simulink model "power_microgrid_v5_battery"  (R2018b)
settings: Solver=ode23tb  StartTime=0.0  StopTime=24*60*60  FixedStep=1/(1000)  MaxStep=60  RelTol=1e-4
PreLoadFcn:
  | load('solar_load_data_24h.mat')
PostLoadFcn:
  | data = xlsread('Domestic_data_all_x3','Sheet1');
  | breakpoints1 = data(2:end,1)'
  | breakpoints2 = data(1,2:end)
  | table_data = data(2:end,2:end)
values from neighbouring files (symbols this model uses):
  SPD_1min = [0 0 0 0 0 0 0 0 0 0 0 0 ... (1441 elements, 1441x1)]    [default_PV_data.mat]
  SPT_1min = [0 60 120 180 240 300 360 420 480 540 600 660 ... (1441 elements, 1441x1)]    [default_PV_data.mat]
libraries: powerlib x155
(part 2 of 5)

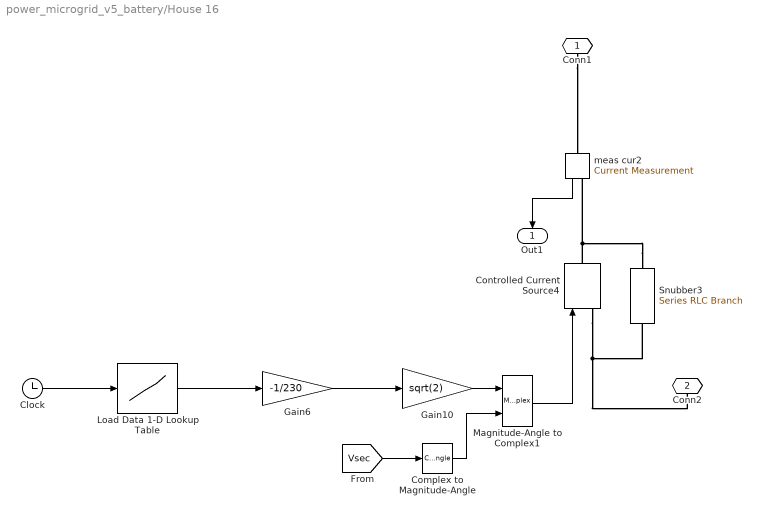
== system power_microgrid_v5_battery/House 16 ==
  Clock : Clock
  Complex to Magnitude-Angle : ComplexToMagnitudeAngle  Output=Angle
  Controlled Current Source4 : powerlib/Electrical Sources/Controlled Current Source  Initialize=on  Source_Type=AC  Amplitude=0  Phase=0  Frequency=50  Measurements=None
      settings: SourceProductName=Simscape Electrical
  Gain10 : Gain  Gain=sqrt(2)
  Gain6 : Gain  Gain=-1/230
  Load Data 1-D Lookup Table : Lookup_n-D  NumberOfTableDimensions=1  BreakpointsForDimension1="[0.00\t600.00\t1200.00\t1800.00\t2400.00\t3000.00\t3600.00\t4200.00\t4800.00\t5400.00\t6000.00\t6600.00\t7200.00\t7800.00\t8400.00\t9000.00\t9600.00\t10200.00\t10800.00\t11400.00\t12000.00\t12600.00\t13200.00\t13800.00\t14400.00\t15000.00\t15600.00\t16200.00\t16800.00\t17400.00\t18000.00\t18600.00\t19200.00\t19800.00\t20400.00\t21000.00\t21600.00\t22200.00\t22800.00\t23400.00\t24000.00\t24600.00\t25200.00\t25800.00\t26400.00\t27000.00\t27600.00\t28200.00\t28800.00\t29400.00\t30000.00\t30600.00\t31200.00\t31800.00\t32400.00\t33000.00\t33600.00\t34200.00\t34800.00\t35400.00\t36000.00\t36600.00\t37200.00\t37800.00\t38400.00\t39000.00\t39600.00\t40200.00\t40800.00\t41400.00\t42000.00\t42600.00\t43200.00\t43800.00\t44400.00\t45000.00\t45600.00\t46200.00\t46800.00\t47400.00\t48000.00\t48600.00\t49200.00\t49800.00\t50400.00\t51000.00\t51600.00\t52200.00\t52800.00\t53400.00\t54000.00\t54600.00\t55200.00\t55800.00\t56400.00\t57000.00\t57600.00\t58200.00\t58800.00\t59400.00\t60000.00\t60600.00\t61200.00\t61800.00\t62400.00\t63000.00\t63600.00\t64200.00\t64800.00\t65400.00\t66000.00\t66600.00\t67200.00\t67800.00\t68400.00\t69000.00\t69600.00\t70200.00\t70800.00\t71400.00\t72000.00\t72600.00\t73200.00\t73800.00\t74400.00\t75000.00\t75600.00\t76200.00\t76800.00\t77400.00\t78000.00\t78600.00\t79200.00\t79800.00\t80400.00\t81000.00\t81600.00\t82200.00\t82800.00\t83400.00\t84000.00\t84600.00\t85200.00\t85800.00\t86400.00]"  BeginIndexSearchUsingPreviousIndexResult=on  Table="[179.5\t163.3\t152.9\t132.5\t118.9\t111.3\t124.6\t103.3\t83.5\t81.2\t85.9\t85.2\t91.9\t95.6\t95.9\t81.8\t83.7\t86.7\t93.8\t81.2\t92.7\t99.4\t112.6\t88.2\t85.6\t78.4\t88.4\t93.9\t86.1\t86.0\t111.7\t143.5\t122.7\t136.8\t142.2\t135.1\t145.6\t141.8\t152.1\t140.3\t167.9\t256.6\t226.1\t263.8\t283.9\t303.3\t279.5\t294.9\t282.3\t288.8\t333.5\t360.9\t421.4\t494.2\t392.5\t439.7\t395.9\t394.4\t364.9\t353.0\t359.1\t370.9\t398.5\t447.4\t344.5\t330.8\t306.8\t331.3\t331.9\t307.6\t371.3\t387.4\t376.6\t360.2\t414.1\t445.1\t411.1\t389.5\t425.2\t340.0\t316.3\t332.8\t352.3\t301.8\t261.8\t298.1\t350.9\t327.8\t296.5\t319.6\t368.4\t327.2\t265.7\t277.9\t292.9\t301.4\t377.9\t336.0\t324.6\t353.8\t389.7\t355.9\t328.4\t325.9\t378.1\t338.0\t379.1\t414.8\t418.1\t464.8\t488.1\t489.1\t485.7\t581.3\t579.7\t526.2\t551.4\t618.6\t628.5\t578.8\t553.3\t481.5\t455.6\t487.9\t507.3\t497.6\t515.4\t510.2\t490.5\t500.5\t494.1\t532.9\t506.5\t466.6\t438.0\t385.4\t381.2\t385.9\t351.7\t371.3\t340.8\t320.2\t277.0\t228.9\t179.5]"  InternalRulePriority=Speed  RndMeth=Simplest  InputSameDT=on
  Magnitude-Angle to Complex1 : MagnitudeAngleToComplex
  Snubber3 : powerlib/Elements/Series RLC Branch  LConnTagsString=__new0  RConnTagsString=__new0  BranchType=R  Resistance=1e6  Inductance=1e-3  SetiL0=off  InitialCurrent=0  Capacitance=1e-6  Setx0=off  InitialVoltage=0  Measurements=None
      settings: SourceProductName=Simscape Electrical
  meas cur2 : powerlib/Measurements/Current Measurement  PhasorSimulation=on  OutputType=Complex  PSBequivalent=0
      settings: SourceProductName=Simscape Electrical
  Conn1 : PMIOPort  Side=Left
  Conn2 : PMIOPort  Port=2  Side=Right
  Out1 : Outport
  wires:
  meas cur2/1 -> Out1/1
  Clock/1 -> Load Data 1-D Lookup Table/1
  Magnitude-Angle to Complex1/1 -> Controlled Current Source4/1
  Load Data 1-D Lookup Table/1 -> Gain6/1
  Complex to Magnitude-Angle/1 -> Magnitude-Angle to Complex1/2
  Gain10/1 -> Magnitude-Angle to Complex1/1
  Gain6/1 -> Gain10/1
  [Vsec] -> Complex to Magnitude-Angle/1
  connections:
  Conn1/RConn1 -- meas cur2/LConn1
  Snubber3/LConn1 -- meas cur2/RConn1 -- Controlled Current Source4/RConn1
  Snubber3/RConn1 -- Controlled Current Source4/LConn1 -- Conn2/RConn1

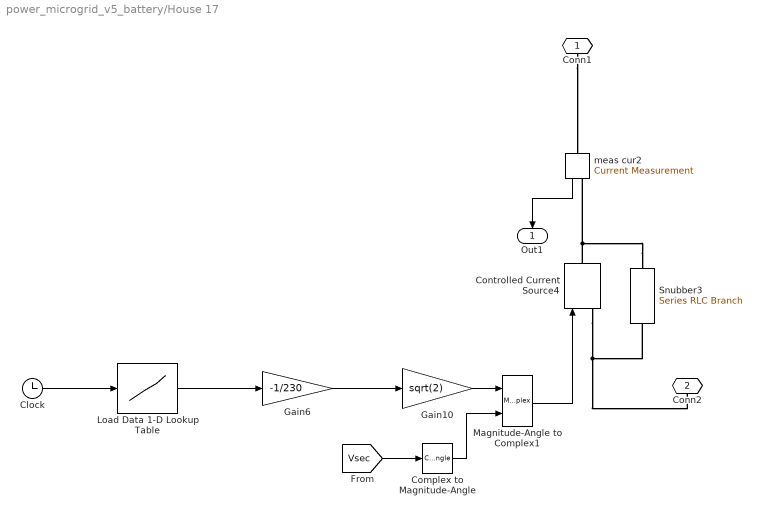
== system power_microgrid_v5_battery/House 17 ==
  Clock : Clock
  Complex to Magnitude-Angle : ComplexToMagnitudeAngle  Output=Angle
  Controlled Current Source4 : powerlib/Electrical Sources/Controlled Current Source  Initialize=on  Source_Type=AC  Amplitude=0  Phase=0  Frequency=50  Measurements=None
      settings: SourceProductName=Simscape Electrical
  Gain10 : Gain  Gain=sqrt(2)
  Gain6 : Gain  Gain=-1/230
  Load Data 1-D Lookup Table : Lookup_n-D  NumberOfTableDimensions=1  BreakpointsForDimension1="[0.00\t600.00\t1200.00\t1800.00\t2400.00\t3000.00\t3600.00\t4200.00\t4800.00\t5400.00\t6000.00\t6600.00\t7200.00\t7800.00\t8400.00\t9000.00\t9600.00\t10200.00\t10800.00\t11400.00\t12000.00\t12600.00\t13200.00\t13800.00\t14400.00\t15000.00\t15600.00\t16200.00\t16800.00\t17400.00\t18000.00\t18600.00\t19200.00\t19800.00\t20400.00\t21000.00\t21600.00\t22200.00\t22800.00\t23400.00\t24000.00\t24600.00\t25200.00\t25800.00\t26400.00\t27000.00\t27600.00\t28200.00\t28800.00\t29400.00\t30000.00\t30600.00\t31200.00\t31800.00\t32400.00\t33000.00\t33600.00\t34200.00\t34800.00\t35400.00\t36000.00\t36600.00\t37200.00\t37800.00\t38400.00\t39000.00\t39600.00\t40200.00\t40800.00\t41400.00\t42000.00\t42600.00\t43200.00\t43800.00\t44400.00\t45000.00\t45600.00\t46200.00\t46800.00\t47400.00\t48000.00\t48600.00\t49200.00\t49800.00\t50400.00\t51000.00\t51600.00\t52200.00\t52800.00\t53400.00\t54000.00\t54600.00\t55200.00\t55800.00\t56400.00\t57000.00\t57600.00\t58200.00\t58800.00\t59400.00\t60000.00\t60600.00\t61200.00\t61800.00\t62400.00\t63000.00\t63600.00\t64200.00\t64800.00\t65400.00\t66000.00\t66600.00\t67200.00\t67800.00\t68400.00\t69000.00\t69600.00\t70200.00\t70800.00\t71400.00\t72000.00\t72600.00\t73200.00\t73800.00\t74400.00\t75000.00\t75600.00\t76200.00\t76800.00\t77400.00\t78000.00\t78600.00\t79200.00\t79800.00\t80400.00\t81000.00\t81600.00\t82200.00\t82800.00\t83400.00\t84000.00\t84600.00\t85200.00\t85800.00\t86400.00]"  BeginIndexSearchUsingPreviousIndexResult=on  Table="[179.5\t163.3\t152.9\t132.5\t118.9\t111.3\t124.6\t103.3\t83.5\t81.2\t85.9\t85.2\t91.9\t95.6\t95.9\t81.8\t83.7\t86.7\t93.8\t81.2\t92.7\t99.4\t112.6\t88.2\t85.6\t78.4\t88.4\t93.9\t86.1\t86.0\t111.7\t143.5\t122.7\t136.8\t142.2\t135.1\t145.6\t141.8\t152.1\t140.3\t167.9\t256.6\t226.1\t263.8\t283.9\t303.3\t279.5\t294.9\t282.3\t288.8\t333.5\t360.9\t421.4\t494.2\t392.5\t439.7\t395.9\t394.4\t364.9\t353.0\t359.1\t370.9\t398.5\t447.4\t344.5\t330.8\t306.8\t331.3\t331.9\t307.6\t371.3\t387.4\t376.6\t360.2\t414.1\t445.1\t411.1\t389.5\t425.2\t340.0\t316.3\t332.8\t352.3\t301.8\t261.8\t298.1\t350.9\t327.8\t296.5\t319.6\t368.4\t327.2\t265.7\t277.9\t292.9\t301.4\t377.9\t336.0\t324.6\t353.8\t389.7\t355.9\t328.4\t325.9\t378.1\t338.0\t379.1\t414.8\t418.1\t464.8\t488.1\t489.1\t485.7\t581.3\t579.7\t526.2\t551.4\t618.6\t628.5\t578.8\t553.3\t481.5\t455.6\t487.9\t507.3\t497.6\t515.4\t510.2\t490.5\t500.5\t494.1\t532.9\t506.5\t466.6\t438.0\t385.4\t381.2\t385.9\t351.7\t371.3\t340.8\t320.2\t277.0\t228.9\t179.5]"  InternalRulePriority=Speed  RndMeth=Simplest  InputSameDT=on
  Magnitude-Angle to Complex1 : MagnitudeAngleToComplex
  Snubber3 : powerlib/Elements/Series RLC Branch  LConnTagsString=__new0  RConnTagsString=__new0  BranchType=R  Resistance=1e6  Inductance=1e-3  SetiL0=off  InitialCurrent=0  Capacitance=1e-6  Setx0=off  InitialVoltage=0  Measurements=None
      settings: SourceProductName=Simscape Electrical
  meas cur2 : powerlib/Measurements/Current Measurement  PhasorSimulation=on  OutputType=Complex  PSBequivalent=0
      settings: SourceProductName=Simscape Electrical
  Conn1 : PMIOPort  Side=Left
  Conn2 : PMIOPort  Port=2  Side=Right
  Out1 : Outport
  wires:
  meas cur2/1 -> Out1/1
  Clock/1 -> Load Data 1-D Lookup Table/1
  Magnitude-Angle to Complex1/1 -> Controlled Current Source4/1
  Load Data 1-D Lookup Table/1 -> Gain6/1
  Complex to Magnitude-Angle/1 -> Magnitude-Angle to Complex1/2
  Gain10/1 -> Magnitude-Angle to Complex1/1
  Gain6/1 -> Gain10/1
  [Vsec] -> Complex to Magnitude-Angle/1
  connections:
  Conn1/RConn1 -- meas cur2/LConn1
  Snubber3/LConn1 -- meas cur2/RConn1 -- Controlled Current Source4/RConn1
  Snubber3/RConn1 -- Controlled Current Source4/LConn1 -- Conn2/RConn1

== system power_microgrid_v5_battery/House 18 ==
  Clock : Clock
  Complex to Magnitude-Angle : ComplexToMagnitudeAngle  Output=Angle
  Controlled Current Source4 : powerlib/Electrical Sources/Controlled Current Source  Initialize=on  Source_Type=AC  Amplitude=0  Phase=0  Frequency=50  Measurements=None
      settings: SourceProductName=Simscape Electrical
  Gain10 : Gain  Gain=sqrt(2)
  Gain6 : Gain  Gain=-1/230
  Load Data 1-D Lookup Table : Lookup_n-D  NumberOfTableDimensions=1  BreakpointsForDimension1="[0.00\t600.00\t1200.00\t1800.00\t2400.00\t3000.00\t3600.00\t4200.00\t4800.00\t5400.00\t6000.00\t6600.00\t7200.00\t7800.00\t8400.00\t9000.00\t9600.00\t10200.00\t10800.00\t11400.00\t12000.00\t12600.00\t13200.00\t13800.00\t14400.00\t15000.00\t15600.00\t16200.00\t16800.00\t17400.00\t18000.00\t18600.00\t19200.00\t19800.00\t20400.00\t21000.00\t21600.00\t22200.00\t22800.00\t23400.00\t24000.00\t24600.00\t25200.00\t25800.00\t26400.00\t27000.00\t27600.00\t28200.00\t28800.00\t29400.00\t30000.00\t30600.00\t31200.00\t31800.00\t32400.00\t33000.00\t33600.00\t34200.00\t34800.00\t35400.00\t36000.00\t36600.00\t37200.00\t37800.00\t38400.00\t39000.00\t39600.00\t40200.00\t40800.00\t41400.00\t42000.00\t42600.00\t43200.00\t43800.00\t44400.00\t45000.00\t45600.00\t46200.00\t46800.00\t47400.00\t48000.00\t48600.00\t49200.00\t49800.00\t50400.00\t51000.00\t51600.00\t52200.00\t52800.00\t53400.00\t54000.00\t54600.00\t55200.00\t55800.00\t56400.00\t57000.00\t57600.00\t58200.00\t58800.00\t59400.00\t60000.00\t60600.00\t61200.00\t61800.00\t62400.00\t63000.00\t63600.00\t64200.00\t64800.00\t65400.00\t66000.00\t66600.00\t67200.00\t67800.00\t68400.00\t69000.00\t69600.00\t70200.00\t70800.00\t71400.00\t72000.00\t72600.00\t73200.00\t73800.00\t74400.00\t75000.00\t75600.00\t76200.00\t76800.00\t77400.00\t78000.00\t78600.00\t79200.00\t79800.00\t80400.00\t81000.00\t81600.00\t82200.00\t82800.00\t83400.00\t84000.00\t84600.00\t85200.00\t85800.00\t86400.00]"  BeginIndexSearchUsingPreviousIndexResult=on  Table="[179.5\t163.3\t152.9\t132.5\t118.9\t111.3\t124.6\t103.3\t83.5\t81.2\t85.9\t85.2\t91.9\t95.6\t95.9\t81.8\t83.7\t86.7\t93.8\t81.2\t92.7\t99.4\t112.6\t88.2\t85.6\t78.4\t88.4\t93.9\t86.1\t86.0\t111.7\t143.5\t122.7\t136.8\t142.2\t135.1\t145.6\t141.8\t152.1\t140.3\t167.9\t256.6\t226.1\t263.8\t283.9\t303.3\t279.5\t294.9\t282.3\t288.8\t333.5\t360.9\t421.4\t494.2\t392.5\t439.7\t395.9\t394.4\t364.9\t353.0\t359.1\t370.9\t398.5\t447.4\t344.5\t330.8\t306.8\t331.3\t331.9\t307.6\t371.3\t387.4\t376.6\t360.2\t414.1\t445.1\t411.1\t389.5\t425.2\t340.0\t316.3\t332.8\t352.3\t301.8\t261.8\t298.1\t350.9\t327.8\t296.5\t319.6\t368.4\t327.2\t265.7\t277.9\t292.9\t301.4\t377.9\t336.0\t324.6\t353.8\t389.7\t355.9\t328.4\t325.9\t378.1\t338.0\t379.1\t414.8\t418.1\t464.8\t488.1\t489.1\t485.7\t581.3\t579.7\t526.2\t551.4\t618.6\t628.5\t578.8\t553.3\t481.5\t455.6\t487.9\t507.3\t497.6\t515.4\t510.2\t490.5\t500.5\t494.1\t532.9\t506.5\t466.6\t438.0\t385.4\t381.2\t385.9\t351.7\t371.3\t340.8\t320.2\t277.0\t228.9\t179.5]"  InternalRulePriority=Speed  RndMeth=Simplest  InputSameDT=on
  Magnitude-Angle to Complex1 : MagnitudeAngleToComplex
  Snubber3 : powerlib/Elements/Series RLC Branch  LConnTagsString=__new0  RConnTagsString=__new0  BranchType=R  Resistance=1e6  Inductance=1e-3  SetiL0=off  InitialCurrent=0  Capacitance=1e-6  Setx0=off  InitialVoltage=0  Measurements=None
      settings: SourceProductName=Simscape Electrical
  meas cur2 : powerlib/Measurements/Current Measurement  PhasorSimulation=on  OutputType=Complex  PSBequivalent=0
      settings: SourceProductName=Simscape Electrical
  Conn1 : PMIOPort  Side=Left
  Conn2 : PMIOPort  Port=2  Side=Right
  Out1 : Outport
  wires:
  meas cur2/1 -> Out1/1
  Clock/1 -> Load Data 1-D Lookup Table/1
  Magnitude-Angle to Complex1/1 -> Controlled Current Source4/1
  Load Data 1-D Lookup Table/1 -> Gain6/1
  Complex to Magnitude-Angle/1 -> Magnitude-Angle to Complex1/2
  Gain10/1 -> Magnitude-Angle to Complex1/1
  Gain6/1 -> Gain10/1
  [Vsec] -> Complex to Magnitude-Angle/1
  connections:
  Conn1/RConn1 -- meas cur2/LConn1
  Snubber3/LConn1 -- meas cur2/RConn1 -- Controlled Current Source4/RConn1
  Snubber3/RConn1 -- Controlled Current Source4/LConn1 -- Conn2/RConn1

== system power_microgrid_v5_battery/House 19 ==
  Clock : Clock
  Complex to Magnitude-Angle : ComplexToMagnitudeAngle  Output=Angle
  Controlled Current Source4 : powerlib/Electrical Sources/Controlled Current Source  Initialize=on  Source_Type=AC  Amplitude=0  Phase=0  Frequency=50  Measurements=None
      settings: SourceProductName=Simscape Electrical
  Gain10 : Gain  Gain=sqrt(2)
  Gain6 : Gain  Gain=-1/230
  Load Data 1-D Lookup Table : Lookup_n-D  NumberOfTableDimensions=1  BreakpointsForDimension1="[0.00\t600.00\t1200.00\t1800.00\t2400.00\t3000.00\t3600.00\t4200.00\t4800.00\t5400.00\t6000.00\t6600.00\t7200.00\t7800.00\t8400.00\t9000.00\t9600.00\t10200.00\t10800.00\t11400.00\t12000.00\t12600.00\t13200.00\t13800.00\t14400.00\t15000.00\t15600.00\t16200.00\t16800.00\t17400.00\t18000.00\t18600.00\t19200.00\t19800.00\t20400.00\t21000.00\t21600.00\t22200.00\t22800.00\t23400.00\t24000.00\t24600.00\t25200.00\t25800.00\t26400.00\t27000.00\t27600.00\t28200.00\t28800.00\t29400.00\t30000.00\t30600.00\t31200.00\t31800.00\t32400.00\t33000.00\t33600.00\t34200.00\t34800.00\t35400.00\t36000.00\t36600.00\t37200.00\t37800.00\t38400.00\t39000.00\t39600.00\t40200.00\t40800.00\t41400.00\t42000.00\t42600.00\t43200.00\t43800.00\t44400.00\t45000.00\t45600.00\t46200.00\t46800.00\t47400.00\t48000.00\t48600.00\t49200.00\t49800.00\t50400.00\t51000.00\t51600.00\t52200.00\t52800.00\t53400.00\t54000.00\t54600.00\t55200.00\t55800.00\t56400.00\t57000.00\t57600.00\t58200.00\t58800.00\t59400.00\t60000.00\t60600.00\t61200.00\t61800.00\t62400.00\t63000.00\t63600.00\t64200.00\t64800.00\t65400.00\t66000.00\t66600.00\t67200.00\t67800.00\t68400.00\t69000.00\t69600.00\t70200.00\t70800.00\t71400.00\t72000.00\t72600.00\t73200.00\t73800.00\t74400.00\t75000.00\t75600.00\t76200.00\t76800.00\t77400.00\t78000.00\t78600.00\t79200.00\t79800.00\t80400.00\t81000.00\t81600.00\t82200.00\t82800.00\t83400.00\t84000.00\t84600.00\t85200.00\t85800.00\t86400.00]"  BeginIndexSearchUsingPreviousIndexResult=on  Table="[179.5\t163.3\t152.9\t132.5\t118.9\t111.3\t124.6\t103.3\t83.5\t81.2\t85.9\t85.2\t91.9\t95.6\t95.9\t81.8\t83.7\t86.7\t93.8\t81.2\t92.7\t99.4\t112.6\t88.2\t85.6\t78.4\t88.4\t93.9\t86.1\t86.0\t111.7\t143.5\t122.7\t136.8\t142.2\t135.1\t145.6\t141.8\t152.1\t140.3\t167.9\t256.6\t226.1\t263.8\t283.9\t303.3\t279.5\t294.9\t282.3\t288.8\t333.5\t360.9\t421.4\t494.2\t392.5\t439.7\t395.9\t394.4\t364.9\t353.0\t359.1\t370.9\t398.5\t447.4\t344.5\t330.8\t306.8\t331.3\t331.9\t307.6\t371.3\t387.4\t376.6\t360.2\t414.1\t445.1\t411.1\t389.5\t425.2\t340.0\t316.3\t332.8\t352.3\t301.8\t261.8\t298.1\t350.9\t327.8\t296.5\t319.6\t368.4\t327.2\t265.7\t277.9\t292.9\t301.4\t377.9\t336.0\t324.6\t353.8\t389.7\t355.9\t328.4\t325.9\t378.1\t338.0\t379.1\t414.8\t418.1\t464.8\t488.1\t489.1\t485.7\t581.3\t579.7\t526.2\t551.4\t618.6\t628.5\t578.8\t553.3\t481.5\t455.6\t487.9\t507.3\t497.6\t515.4\t510.2\t490.5\t500.5\t494.1\t532.9\t506.5\t466.6\t438.0\t385.4\t381.2\t385.9\t351.7\t371.3\t340.8\t320.2\t277.0\t228.9\t179.5]"  InternalRulePriority=Speed  RndMeth=Simplest  InputSameDT=on
  Magnitude-Angle to Complex1 : MagnitudeAngleToComplex
  Snubber3 : powerlib/Elements/Series RLC Branch  LConnTagsString=__new0  RConnTagsString=__new0  BranchType=R  Resistance=1e6  Inductance=1e-3  SetiL0=off  InitialCurrent=0  Capacitance=1e-6  Setx0=off  InitialVoltage=0  Measurements=None
      settings: SourceProductName=Simscape Electrical
  meas cur2 : powerlib/Measurements/Current Measurement  PhasorSimulation=on  OutputType=Complex  PSBequivalent=0
      settings: SourceProductName=Simscape Electrical
  Conn1 : PMIOPort  Side=Left
  Conn2 : PMIOPort  Port=2  Side=Right
  Out1 : Outport
  wires:
  meas cur2/1 -> Out1/1
  Clock/1 -> Load Data 1-D Lookup Table/1
  Magnitude-Angle to Complex1/1 -> Controlled Current Source4/1
  Load Data 1-D Lookup Table/1 -> Gain6/1
  Complex to Magnitude-Angle/1 -> Magnitude-Angle to Complex1/2
  Gain10/1 -> Magnitude-Angle to Complex1/1
  Gain6/1 -> Gain10/1
  [Vsec] -> Complex to Magnitude-Angle/1
  connections:
  Conn1/RConn1 -- meas cur2/LConn1
  Snubber3/LConn1 -- meas cur2/RConn1 -- Controlled Current Source4/RConn1
  Snubber3/RConn1 -- Controlled Current Source4/LConn1 -- Conn2/RConn1

== system power_microgrid_v5_battery/House 2 ==
  Clock : Clock
  Complex to Magnitude-Angle : ComplexToMagnitudeAngle  Output=Angle
  Controlled Current Source4 : powerlib/Electrical Sources/Controlled Current Source  Initialize=on  Source_Type=AC  Amplitude=0  Phase=0  Frequency=50  Measurements=None
      settings: SourceProductName=Simscape Electrical
  Gain10 : Gain  Gain=sqrt(2)
  Gain6 : Gain  Gain=-1/230
  Load Data 1-D Lookup Table : Lookup_n-D  NumberOfTableDimensions=1  BreakpointsForDimension1="[0.00\t600.00\t1200.00\t1800.00\t2400.00\t3000.00\t3600.00\t4200.00\t4800.00\t5400.00\t6000.00\t6600.00\t7200.00\t7800.00\t8400.00\t9000.00\t9600.00\t10200.00\t10800.00\t11400.00\t12000.00\t12600.00\t13200.00\t13800.00\t14400.00\t15000.00\t15600.00\t16200.00\t16800.00\t17400.00\t18000.00\t18600.00\t19200.00\t19800.00\t20400.00\t21000.00\t21600.00\t22200.00\t22800.00\t23400.00\t24000.00\t24600.00\t25200.00\t25800.00\t26400.00\t27000.00\t27600.00\t28200.00\t28800.00\t29400.00\t30000.00\t30600.00\t31200.00\t31800.00\t32400.00\t33000.00\t33600.00\t34200.00\t34800.00\t35400.00\t36000.00\t36600.00\t37200.00\t37800.00\t38400.00\t39000.00\t39600.00\t40200.00\t40800.00\t41400.00\t42000.00\t42600.00\t43200.00\t43800.00\t44400.00\t45000.00\t45600.00\t46200.00\t46800.00\t47400.00\t48000.00\t48600.00\t49200.00\t49800.00\t50400.00\t51000.00\t51600.00\t52200.00\t52800.00\t53400.00\t54000.00\t54600.00\t55200.00\t55800.00\t56400.00\t57000.00\t57600.00\t58200.00\t58800.00\t59400.00\t60000.00\t60600.00\t61200.00\t61800.00\t62400.00\t63000.00\t63600.00\t64200.00\t64800.00\t65400.00\t66000.00\t66600.00\t67200.00\t67800.00\t68400.00\t69000.00\t69600.00\t70200.00\t70800.00\t71400.00\t72000.00\t72600.00\t73200.00\t73800.00\t74400.00\t75000.00\t75600.00\t76200.00\t76800.00\t77400.00\t78000.00\t78600.00\t79200.00\t79800.00\t80400.00\t81000.00\t81600.00\t82200.00\t82800.00\t83400.00\t84000.00\t84600.00\t85200.00\t85800.00\t86400.00]"  BeginIndexSearchUsingPreviousIndexResult=on  Table="[179.5\t163.3\t152.9\t132.5\t118.9\t111.3\t124.6\t103.3\t83.5\t81.2\t85.9\t85.2\t91.9\t95.6\t95.9\t81.8\t83.7\t86.7\t93.8\t81.2\t92.7\t99.4\t112.6\t88.2\t85.6\t78.4\t88.4\t93.9\t86.1\t86.0\t111.7\t143.5\t122.7\t136.8\t142.2\t135.1\t145.6\t141.8\t152.1\t140.3\t167.9\t256.6\t226.1\t263.8\t283.9\t303.3\t279.5\t294.9\t282.3\t288.8\t333.5\t360.9\t421.4\t494.2\t392.5\t439.7\t395.9\t394.4\t364.9\t353.0\t359.1\t370.9\t398.5\t447.4\t344.5\t330.8\t306.8\t331.3\t331.9\t307.6\t371.3\t387.4\t376.6\t360.2\t414.1\t445.1\t411.1\t389.5\t425.2\t340.0\t316.3\t332.8\t352.3\t301.8\t261.8\t298.1\t350.9\t327.8\t296.5\t319.6\t368.4\t327.2\t265.7\t277.9\t292.9\t301.4\t377.9\t336.0\t324.6\t353.8\t389.7\t355.9\t328.4\t325.9\t378.1\t338.0\t379.1\t414.8\t418.1\t464.8\t488.1\t489.1\t485.7\t581.3\t579.7\t526.2\t551.4\t618.6\t628.5\t578.8\t553.3\t481.5\t455.6\t487.9\t507.3\t497.6\t515.4\t510.2\t490.5\t500.5\t494.1\t532.9\t506.5\t466.6\t438.0\t385.4\t381.2\t385.9\t351.7\t371.3\t340.8\t320.2\t277.0\t228.9\t179.5]"  InternalRulePriority=Speed  RndMeth=Simplest  InputSameDT=on
  Magnitude-Angle to Complex1 : MagnitudeAngleToComplex
  Snubber3 : powerlib/Elements/Series RLC Branch  LConnTagsString=__new0  RConnTagsString=__new0  BranchType=R  Resistance=1e6  Inductance=1e-3  SetiL0=off  InitialCurrent=0  Capacitance=1e-6  Setx0=off  InitialVoltage=0  Measurements=None
      settings: SourceProductName=Simscape Electrical
  meas cur2 : powerlib/Measurements/Current Measurement  PhasorSimulation=on  OutputType=Complex  PSBequivalent=0
      settings: SourceProductName=Simscape Electrical
  Conn1 : PMIOPort  Side=Left
  Conn2 : PMIOPort  Port=2  Side=Right
  Out1 : Outport
  wires:
  meas cur2/1 -> Out1/1
  Clock/1 -> Load Data 1-D Lookup Table/1
  Magnitude-Angle to Complex1/1 -> Controlled Current Source4/1
  Load Data 1-D Lookup Table/1 -> Gain6/1
  Complex to Magnitude-Angle/1 -> Magnitude-Angle to Complex1/2
  Gain10/1 -> Magnitude-Angle to Complex1/1
  Gain6/1 -> Gain10/1
  [Vsec] -> Complex to Magnitude-Angle/1
  connections:
  Conn1/RConn1 -- meas cur2/LConn1
  Snubber3/LConn1 -- meas cur2/RConn1 -- Controlled Current Source4/RConn1
  Snubber3/RConn1 -- Controlled Current Source4/LConn1 -- Conn2/RConn1

== system power_microgrid_v5_battery/House 20 ==
  Clock : Clock
  Complex to Magnitude-Angle : ComplexToMagnitudeAngle  Output=Angle
  Controlled Current Source4 : powerlib/Electrical Sources/Controlled Current Source  Initialize=on  Source_Type=AC  Amplitude=0  Phase=0  Frequency=50  Measurements=None
      settings: SourceProductName=Simscape Electrical
  Gain10 : Gain  Gain=sqrt(2)
  Gain6 : Gain  Gain=-1/230
  Load Data 1-D Lookup Table : Lookup_n-D  NumberOfTableDimensions=1  BreakpointsForDimension1="[0.00\t600.00\t1200.00\t1800.00\t2400.00\t3000.00\t3600.00\t4200.00\t4800.00\t5400.00\t6000.00\t6600.00\t7200.00\t7800.00\t8400.00\t9000.00\t9600.00\t10200.00\t10800.00\t11400.00\t12000.00\t12600.00\t13200.00\t13800.00\t14400.00\t15000.00\t15600.00\t16200.00\t16800.00\t17400.00\t18000.00\t18600.00\t19200.00\t19800.00\t20400.00\t21000.00\t21600.00\t22200.00\t22800.00\t23400.00\t24000.00\t24600.00\t25200.00\t25800.00\t26400.00\t27000.00\t27600.00\t28200.00\t28800.00\t29400.00\t30000.00\t30600.00\t31200.00\t31800.00\t32400.00\t33000.00\t33600.00\t34200.00\t34800.00\t35400.00\t36000.00\t36600.00\t37200.00\t37800.00\t38400.00\t39000.00\t39600.00\t40200.00\t40800.00\t41400.00\t42000.00\t42600.00\t43200.00\t43800.00\t44400.00\t45000.00\t45600.00\t46200.00\t46800.00\t47400.00\t48000.00\t48600.00\t49200.00\t49800.00\t50400.00\t51000.00\t51600.00\t52200.00\t52800.00\t53400.00\t54000.00\t54600.00\t55200.00\t55800.00\t56400.00\t57000.00\t57600.00\t58200.00\t58800.00\t59400.00\t60000.00\t60600.00\t61200.00\t61800.00\t62400.00\t63000.00\t63600.00\t64200.00\t64800.00\t65400.00\t66000.00\t66600.00\t67200.00\t67800.00\t68400.00\t69000.00\t69600.00\t70200.00\t70800.00\t71400.00\t72000.00\t72600.00\t73200.00\t73800.00\t74400.00\t75000.00\t75600.00\t76200.00\t76800.00\t77400.00\t78000.00\t78600.00\t79200.00\t79800.00\t80400.00\t81000.00\t81600.00\t82200.00\t82800.00\t83400.00\t84000.00\t84600.00\t85200.00\t85800.00\t86400.00]"  BeginIndexSearchUsingPreviousIndexResult=on  Table="[176.6\t168.8\t171.0\t162.4\t139.2\t135.7\t136.1\t126.4\t115.3\t119.1\t120.9\t112.9\t108.8\t108.4\t108.6\t115.7\t109.1\t110.1\t104.3\t102.4\t107.1\t108.6\t105.0\t101.7\t101.0\t100.5\t104.1\t105.9\t110.2\t113.1\t112.9\t122.1\t109.2\t120.3\t118.6\t122.6\t124.2\t134.1\t162.8\t189.0\t309.3\t319.3\t364.8\t346.9\t417.0\t276.3\t256.5\t386.4\t343.0\t281.6\t284.9\t297.7\t367.6\t344.5\t340.2\t401.7\t337.5\t290.1\t263.4\t283.0\t256.4\t264.4\t333.9\t339.9\t228.2\t258.4\t286.7\t337.2\t345.7\t283.4\t271.5\t301.9\t315.2\t222.7\t260.5\t314.4\t276.6\t251.0\t286.5\t277.6\t337.1\t293.1\t272.6\t264.0\t234.7\t266.6\t312.4\t300.4\t272.7\t275.3\t328.8\t303.7\t296.9\t271.1\t276.5\t287.6\t336.9\t310.5\t308.1\t352.7\t369.3\t416.5\t395.6\t425.3\t391.6\t343.9\t385.2\t411.7\t419.9\t433.6\t448.9\t437.5\t456.3\t466.2\t475.8\t478.2\t421.9\t455.4\t432.7\t434.7\t414.2\t380.6\t376.3\t380.7\t364.6\t365.6\t376.3\t400.0\t428.4\t382.9\t369.3\t440.8\t388.9\t372.9\t362.3\t328.6\t292.7\t286.7\t266.4\t263.2\t248.0\t239.3\t218.5\t190.8\t176.6]"  InternalRulePriority=Speed  RndMeth=Simplest  InputSameDT=on
  Magnitude-Angle to Complex1 : MagnitudeAngleToComplex
  Snubber3 : powerlib/Elements/Series RLC Branch  LConnTagsString=__new0  RConnTagsString=__new0  BranchType=R  Resistance=1e6  Inductance=1e-3  SetiL0=off  InitialCurrent=0  Capacitance=1e-6  Setx0=off  InitialVoltage=0  Measurements=None
      settings: SourceProductName=Simscape Electrical
  meas cur2 : powerlib/Measurements/Current Measurement  PhasorSimulation=on  OutputType=Complex  PSBequivalent=0
      settings: SourceProductName=Simscape Electrical
  Conn1 : PMIOPort  Side=Left
  Conn2 : PMIOPort  Port=2  Side=Right
  Out1 : Outport
  wires:
  Magnitude-Angle to Complex1/1 -> Controlled Current Source4/1
  meas cur2/1 -> Out1/1
  Clock/1 -> Load Data 1-D Lookup Table/1
  Load Data 1-D Lookup Table/1 -> Gain6/1
  [Vsec] -> Complex to Magnitude-Angle/1
  Gain6/1 -> Gain10/1
  Gain10/1 -> Magnitude-Angle to Complex1/1
  Complex to Magnitude-Angle/1 -> Magnitude-Angle to Complex1/2
  connections:
  meas cur2/LConn1 -- Conn1/RConn1
  Snubber3/LConn1 -- Controlled Current Source4/RConn1 -- meas cur2/RConn1
  Snubber3/RConn1 -- Controlled Current Source4/LConn1 -- Conn2/RConn1

== system power_microgrid_v5_battery/House 21 ==
  Clock : Clock
  Complex to Magnitude-Angle : ComplexToMagnitudeAngle  Output=Angle
  Controlled Current Source4 : powerlib/Electrical Sources/Controlled Current Source  Initialize=on  Source_Type=AC  Amplitude=0  Phase=0  Frequency=50  Measurements=None
      settings: SourceProductName=Simscape Electrical
  Gain10 : Gain  Gain=sqrt(2)
  Gain6 : Gain  Gain=-1/230
  Load Data 1-D Lookup Table : Lookup_n-D  NumberOfTableDimensions=1  BreakpointsForDimension1="[0.00\t600.00\t1200.00\t1800.00\t2400.00\t3000.00\t3600.00\t4200.00\t4800.00\t5400.00\t6000.00\t6600.00\t7200.00\t7800.00\t8400.00\t9000.00\t9600.00\t10200.00\t10800.00\t11400.00\t12000.00\t12600.00\t13200.00\t13800.00\t14400.00\t15000.00\t15600.00\t16200.00\t16800.00\t17400.00\t18000.00\t18600.00\t19200.00\t19800.00\t20400.00\t21000.00\t21600.00\t22200.00\t22800.00\t23400.00\t24000.00\t24600.00\t25200.00\t25800.00\t26400.00\t27000.00\t27600.00\t28200.00\t28800.00\t29400.00\t30000.00\t30600.00\t31200.00\t31800.00\t32400.00\t33000.00\t33600.00\t34200.00\t34800.00\t35400.00\t36000.00\t36600.00\t37200.00\t37800.00\t38400.00\t39000.00\t39600.00\t40200.00\t40800.00\t41400.00\t42000.00\t42600.00\t43200.00\t43800.00\t44400.00\t45000.00\t45600.00\t46200.00\t46800.00\t47400.00\t48000.00\t48600.00\t49200.00\t49800.00\t50400.00\t51000.00\t51600.00\t52200.00\t52800.00\t53400.00\t54000.00\t54600.00\t55200.00\t55800.00\t56400.00\t57000.00\t57600.00\t58200.00\t58800.00\t59400.00\t60000.00\t60600.00\t61200.00\t61800.00\t62400.00\t63000.00\t63600.00\t64200.00\t64800.00\t65400.00\t66000.00\t66600.00\t67200.00\t67800.00\t68400.00\t69000.00\t69600.00\t70200.00\t70800.00\t71400.00\t72000.00\t72600.00\t73200.00\t73800.00\t74400.00\t75000.00\t75600.00\t76200.00\t76800.00\t77400.00\t78000.00\t78600.00\t79200.00\t79800.00\t80400.00\t81000.00\t81600.00\t82200.00\t82800.00\t83400.00\t84000.00\t84600.00\t85200.00\t85800.00\t86400.00]"  BeginIndexSearchUsingPreviousIndexResult=on  Table="[176.6\t168.8\t171.0\t162.4\t139.2\t135.7\t136.1\t126.4\t115.3\t119.1\t120.9\t112.9\t108.8\t108.4\t108.6\t115.7\t109.1\t110.1\t104.3\t102.4\t107.1\t108.6\t105.0\t101.7\t101.0\t100.5\t104.1\t105.9\t110.2\t113.1\t112.9\t122.1\t109.2\t120.3\t118.6\t122.6\t124.2\t134.1\t162.8\t189.0\t309.3\t319.3\t364.8\t346.9\t417.0\t276.3\t256.5\t386.4\t343.0\t281.6\t284.9\t297.7\t367.6\t344.5\t340.2\t401.7\t337.5\t290.1\t263.4\t283.0\t256.4\t264.4\t333.9\t339.9\t228.2\t258.4\t286.7\t337.2\t345.7\t283.4\t271.5\t301.9\t315.2\t222.7\t260.5\t314.4\t276.6\t251.0\t286.5\t277.6\t337.1\t293.1\t272.6\t264.0\t234.7\t266.6\t312.4\t300.4\t272.7\t275.3\t328.8\t303.7\t296.9\t271.1\t276.5\t287.6\t336.9\t310.5\t308.1\t352.7\t369.3\t416.5\t395.6\t425.3\t391.6\t343.9\t385.2\t411.7\t419.9\t433.6\t448.9\t437.5\t456.3\t466.2\t475.8\t478.2\t421.9\t455.4\t432.7\t434.7\t414.2\t380.6\t376.3\t380.7\t364.6\t365.6\t376.3\t400.0\t428.4\t382.9\t369.3\t440.8\t388.9\t372.9\t362.3\t328.6\t292.7\t286.7\t266.4\t263.2\t248.0\t239.3\t218.5\t190.8\t176.6]"  InternalRulePriority=Speed  RndMeth=Simplest  InputSameDT=on
  Magnitude-Angle to Complex1 : MagnitudeAngleToComplex
  Snubber3 : powerlib/Elements/Series RLC Branch  LConnTagsString=__new0  RConnTagsString=__new0  BranchType=R  Resistance=1e6  Inductance=1e-3  SetiL0=off  InitialCurrent=0  Capacitance=1e-6  Setx0=off  InitialVoltage=0  Measurements=None
      settings: SourceProductName=Simscape Electrical
  meas cur2 : powerlib/Measurements/Current Measurement  PhasorSimulation=on  OutputType=Complex  PSBequivalent=0
      settings: SourceProductName=Simscape Electrical
  Conn1 : PMIOPort  Side=Left
  Conn2 : PMIOPort  Port=2  Side=Right
  Out1 : Outport
  wires:
  Magnitude-Angle to Complex1/1 -> Controlled Current Source4/1
  meas cur2/1 -> Out1/1
  Clock/1 -> Load Data 1-D Lookup Table/1
  Load Data 1-D Lookup Table/1 -> Gain6/1
  [Vsec] -> Complex to Magnitude-Angle/1
  Gain6/1 -> Gain10/1
  Gain10/1 -> Magnitude-Angle to Complex1/1
  Complex to Magnitude-Angle/1 -> Magnitude-Angle to Complex1/2
  connections:
  meas cur2/LConn1 -- Conn1/RConn1
  Snubber3/LConn1 -- Controlled Current Source4/RConn1 -- meas cur2/RConn1
  Snubber3/RConn1 -- Controlled Current Source4/LConn1 -- Conn2/RConn1

== system power_microgrid_v5_battery/House 22 ==
  Clock : Clock
  Complex to Magnitude-Angle : ComplexToMagnitudeAngle  Output=Angle
  Controlled Current Source4 : powerlib/Electrical Sources/Controlled Current Source  Initialize=on  Source_Type=AC  Amplitude=0  Phase=0  Frequency=50  Measurements=None
      settings: SourceProductName=Simscape Electrical
  Gain10 : Gain  Gain=sqrt(2)
  Gain6 : Gain  Gain=-1/230
  Load Data 1-D Lookup Table : Lookup_n-D  NumberOfTableDimensions=1  BreakpointsForDimension1="[0.00\t600.00\t1200.00\t1800.00\t2400.00\t3000.00\t3600.00\t4200.00\t4800.00\t5400.00\t6000.00\t6600.00\t7200.00\t7800.00\t8400.00\t9000.00\t9600.00\t10200.00\t10800.00\t11400.00\t12000.00\t12600.00\t13200.00\t13800.00\t14400.00\t15000.00\t15600.00\t16200.00\t16800.00\t17400.00\t18000.00\t18600.00\t19200.00\t19800.00\t20400.00\t21000.00\t21600.00\t22200.00\t22800.00\t23400.00\t24000.00\t24600.00\t25200.00\t25800.00\t26400.00\t27000.00\t27600.00\t28200.00\t28800.00\t29400.00\t30000.00\t30600.00\t31200.00\t31800.00\t32400.00\t33000.00\t33600.00\t34200.00\t34800.00\t35400.00\t36000.00\t36600.00\t37200.00\t37800.00\t38400.00\t39000.00\t39600.00\t40200.00\t40800.00\t41400.00\t42000.00\t42600.00\t43200.00\t43800.00\t44400.00\t45000.00\t45600.00\t46200.00\t46800.00\t47400.00\t48000.00\t48600.00\t49200.00\t49800.00\t50400.00\t51000.00\t51600.00\t52200.00\t52800.00\t53400.00\t54000.00\t54600.00\t55200.00\t55800.00\t56400.00\t57000.00\t57600.00\t58200.00\t58800.00\t59400.00\t60000.00\t60600.00\t61200.00\t61800.00\t62400.00\t63000.00\t63600.00\t64200.00\t64800.00\t65400.00\t66000.00\t66600.00\t67200.00\t67800.00\t68400.00\t69000.00\t69600.00\t70200.00\t70800.00\t71400.00\t72000.00\t72600.00\t73200.00\t73800.00\t74400.00\t75000.00\t75600.00\t76200.00\t76800.00\t77400.00\t78000.00\t78600.00\t79200.00\t79800.00\t80400.00\t81000.00\t81600.00\t82200.00\t82800.00\t83400.00\t84000.00\t84600.00\t85200.00\t85800.00\t86400.00]"  BeginIndexSearchUsingPreviousIndexResult=on  Table="[176.6\t168.8\t171.0\t162.4\t139.2\t135.7\t136.1\t126.4\t115.3\t119.1\t120.9\t112.9\t108.8\t108.4\t108.6\t115.7\t109.1\t110.1\t104.3\t102.4\t107.1\t108.6\t105.0\t101.7\t101.0\t100.5\t104.1\t105.9\t110.2\t113.1\t112.9\t122.1\t109.2\t120.3\t118.6\t122.6\t124.2\t134.1\t162.8\t189.0\t309.3\t319.3\t364.8\t346.9\t417.0\t276.3\t256.5\t386.4\t343.0\t281.6\t284.9\t297.7\t367.6\t344.5\t340.2\t401.7\t337.5\t290.1\t263.4\t283.0\t256.4\t264.4\t333.9\t339.9\t228.2\t258.4\t286.7\t337.2\t345.7\t283.4\t271.5\t301.9\t315.2\t222.7\t260.5\t314.4\t276.6\t251.0\t286.5\t277.6\t337.1\t293.1\t272.6\t264.0\t234.7\t266.6\t312.4\t300.4\t272.7\t275.3\t328.8\t303.7\t296.9\t271.1\t276.5\t287.6\t336.9\t310.5\t308.1\t352.7\t369.3\t416.5\t395.6\t425.3\t391.6\t343.9\t385.2\t411.7\t419.9\t433.6\t448.9\t437.5\t456.3\t466.2\t475.8\t478.2\t421.9\t455.4\t432.7\t434.7\t414.2\t380.6\t376.3\t380.7\t364.6\t365.6\t376.3\t400.0\t428.4\t382.9\t369.3\t440.8\t388.9\t372.9\t362.3\t328.6\t292.7\t286.7\t266.4\t263.2\t248.0\t239.3\t218.5\t190.8\t176.6]"  InternalRulePriority=Speed  RndMeth=Simplest  InputSameDT=on
  Magnitude-Angle to Complex1 : MagnitudeAngleToComplex
  Snubber3 : powerlib/Elements/Series RLC Branch  LConnTagsString=__new0  RConnTagsString=__new0  BranchType=R  Resistance=1e6  Inductance=1e-3  SetiL0=off  InitialCurrent=0  Capacitance=1e-6  Setx0=off  InitialVoltage=0  Measurements=None
      settings: SourceProductName=Simscape Electrical
  meas cur2 : powerlib/Measurements/Current Measurement  PhasorSimulation=on  OutputType=Complex  PSBequivalent=0
      settings: SourceProductName=Simscape Electrical
  Conn1 : PMIOPort  Side=Left
  Conn2 : PMIOPort  Port=2  Side=Right
  Out1 : Outport
  wires:
  meas cur2/1 -> Out1/1
  Clock/1 -> Load Data 1-D Lookup Table/1
  Magnitude-Angle to Complex1/1 -> Controlled Current Source4/1
  Load Data 1-D Lookup Table/1 -> Gain6/1
  Complex to Magnitude-Angle/1 -> Magnitude-Angle to Complex1/2
  Gain10/1 -> Magnitude-Angle to Complex1/1
  Gain6/1 -> Gain10/1
  [Vsec] -> Complex to Magnitude-Angle/1
  connections:
  Conn1/RConn1 -- meas cur2/LConn1
  Snubber3/LConn1 -- meas cur2/RConn1 -- Controlled Current Source4/RConn1
  Snubber3/RConn1 -- Controlled Current Source4/LConn1 -- Conn2/RConn1

== system power_microgrid_v5_battery/House 23 ==
  Clock : Clock
  Complex to Magnitude-Angle : ComplexToMagnitudeAngle  Output=Angle
  Controlled Current Source4 : powerlib/Electrical Sources/Controlled Current Source  Initialize=on  Source_Type=AC  Amplitude=0  Phase=0  Frequency=50  Measurements=None
      settings: SourceProductName=Simscape Electrical
  Gain10 : Gain  Gain=sqrt(2)
  Gain6 : Gain  Gain=-1/230
  Load Data 1-D Lookup Table : Lookup_n-D  NumberOfTableDimensions=1  BreakpointsForDimension1="[0.00\t600.00\t1200.00\t1800.00\t2400.00\t3000.00\t3600.00\t4200.00\t4800.00\t5400.00\t6000.00\t6600.00\t7200.00\t7800.00\t8400.00\t9000.00\t9600.00\t10200.00\t10800.00\t11400.00\t12000.00\t12600.00\t13200.00\t13800.00\t14400.00\t15000.00\t15600.00\t16200.00\t16800.00\t17400.00\t18000.00\t18600.00\t19200.00\t19800.00\t20400.00\t21000.00\t21600.00\t22200.00\t22800.00\t23400.00\t24000.00\t24600.00\t25200.00\t25800.00\t26400.00\t27000.00\t27600.00\t28200.00\t28800.00\t29400.00\t30000.00\t30600.00\t31200.00\t31800.00\t32400.00\t33000.00\t33600.00\t34200.00\t34800.00\t35400.00\t36000.00\t36600.00\t37200.00\t37800.00\t38400.00\t39000.00\t39600.00\t40200.00\t40800.00\t41400.00\t42000.00\t42600.00\t43200.00\t43800.00\t44400.00\t45000.00\t45600.00\t46200.00\t46800.00\t47400.00\t48000.00\t48600.00\t49200.00\t49800.00\t50400.00\t51000.00\t51600.00\t52200.00\t52800.00\t53400.00\t54000.00\t54600.00\t55200.00\t55800.00\t56400.00\t57000.00\t57600.00\t58200.00\t58800.00\t59400.00\t60000.00\t60600.00\t61200.00\t61800.00\t62400.00\t63000.00\t63600.00\t64200.00\t64800.00\t65400.00\t66000.00\t66600.00\t67200.00\t67800.00\t68400.00\t69000.00\t69600.00\t70200.00\t70800.00\t71400.00\t72000.00\t72600.00\t73200.00\t73800.00\t74400.00\t75000.00\t75600.00\t76200.00\t76800.00\t77400.00\t78000.00\t78600.00\t79200.00\t79800.00\t80400.00\t81000.00\t81600.00\t82200.00\t82800.00\t83400.00\t84000.00\t84600.00\t85200.00\t85800.00\t86400.00]"  BeginIndexSearchUsingPreviousIndexResult=on  Table="[176.6\t168.8\t171.0\t162.4\t139.2\t135.7\t136.1\t126.4\t115.3\t119.1\t120.9\t112.9\t108.8\t108.4\t108.6\t115.7\t109.1\t110.1\t104.3\t102.4\t107.1\t108.6\t105.0\t101.7\t101.0\t100.5\t104.1\t105.9\t110.2\t113.1\t112.9\t122.1\t109.2\t120.3\t118.6\t122.6\t124.2\t134.1\t162.8\t189.0\t309.3\t319.3\t364.8\t346.9\t417.0\t276.3\t256.5\t386.4\t343.0\t281.6\t284.9\t297.7\t367.6\t344.5\t340.2\t401.7\t337.5\t290.1\t263.4\t283.0\t256.4\t264.4\t333.9\t339.9\t228.2\t258.4\t286.7\t337.2\t345.7\t283.4\t271.5\t301.9\t315.2\t222.7\t260.5\t314.4\t276.6\t251.0\t286.5\t277.6\t337.1\t293.1\t272.6\t264.0\t234.7\t266.6\t312.4\t300.4\t272.7\t275.3\t328.8\t303.7\t296.9\t271.1\t276.5\t287.6\t336.9\t310.5\t308.1\t352.7\t369.3\t416.5\t395.6\t425.3\t391.6\t343.9\t385.2\t411.7\t419.9\t433.6\t448.9\t437.5\t456.3\t466.2\t475.8\t478.2\t421.9\t455.4\t432.7\t434.7\t414.2\t380.6\t376.3\t380.7\t364.6\t365.6\t376.3\t400.0\t428.4\t382.9\t369.3\t440.8\t388.9\t372.9\t362.3\t328.6\t292.7\t286.7\t266.4\t263.2\t248.0\t239.3\t218.5\t190.8\t176.6]"  InternalRulePriority=Speed  RndMeth=Simplest  InputSameDT=on
  Magnitude-Angle to Complex1 : MagnitudeAngleToComplex
  Snubber3 : powerlib/Elements/Series RLC Branch  LConnTagsString=__new0  RConnTagsString=__new0  BranchType=R  Resistance=1e6  Inductance=1e-3  SetiL0=off  InitialCurrent=0  Capacitance=1e-6  Setx0=off  InitialVoltage=0  Measurements=None
      settings: SourceProductName=Simscape Electrical
  meas cur2 : powerlib/Measurements/Current Measurement  PhasorSimulation=on  OutputType=Complex  PSBequivalent=0
      settings: SourceProductName=Simscape Electrical
  Conn1 : PMIOPort  Side=Left
  Conn2 : PMIOPort  Port=2  Side=Right
  Out1 : Outport
  wires:
  Magnitude-Angle to Complex1/1 -> Controlled Current Source4/1
  meas cur2/1 -> Out1/1
  Clock/1 -> Load Data 1-D Lookup Table/1
  Load Data 1-D Lookup Table/1 -> Gain6/1
  [Vsec] -> Complex to Magnitude-Angle/1
  Gain6/1 -> Gain10/1
  Gain10/1 -> Magnitude-Angle to Complex1/1
  Complex to Magnitude-Angle/1 -> Magnitude-Angle to Complex1/2
  connections:
  meas cur2/LConn1 -- Conn1/RConn1
  Snubber3/LConn1 -- Controlled Current Source4/RConn1 -- meas cur2/RConn1
  Snubber3/RConn1 -- Controlled Current Source4/LConn1 -- Conn2/RConn1

== system power_microgrid_v5_battery/House 24 ==
  Clock : Clock
  Complex to Magnitude-Angle : ComplexToMagnitudeAngle  Output=Angle
  Controlled Current Source4 : powerlib/Electrical Sources/Controlled Current Source  Initialize=on  Source_Type=AC  Amplitude=0  Phase=0  Frequency=50  Measurements=None
      settings: SourceProductName=Simscape Electrical
  Gain10 : Gain  Gain=sqrt(2)
  Gain6 : Gain  Gain=-1/230
  Load Data 1-D Lookup Table : Lookup_n-D  NumberOfTableDimensions=1  BreakpointsForDimension1="[0.00\t600.00\t1200.00\t1800.00\t2400.00\t3000.00\t3600.00\t4200.00\t4800.00\t5400.00\t6000.00\t6600.00\t7200.00\t7800.00\t8400.00\t9000.00\t9600.00\t10200.00\t10800.00\t11400.00\t12000.00\t12600.00\t13200.00\t13800.00\t14400.00\t15000.00\t15600.00\t16200.00\t16800.00\t17400.00\t18000.00\t18600.00\t19200.00\t19800.00\t20400.00\t21000.00\t21600.00\t22200.00\t22800.00\t23400.00\t24000.00\t24600.00\t25200.00\t25800.00\t26400.00\t27000.00\t27600.00\t28200.00\t28800.00\t29400.00\t30000.00\t30600.00\t31200.00\t31800.00\t32400.00\t33000.00\t33600.00\t34200.00\t34800.00\t35400.00\t36000.00\t36600.00\t37200.00\t37800.00\t38400.00\t39000.00\t39600.00\t40200.00\t40800.00\t41400.00\t42000.00\t42600.00\t43200.00\t43800.00\t44400.00\t45000.00\t45600.00\t46200.00\t46800.00\t47400.00\t48000.00\t48600.00\t49200.00\t49800.00\t50400.00\t51000.00\t51600.00\t52200.00\t52800.00\t53400.00\t54000.00\t54600.00\t55200.00\t55800.00\t56400.00\t57000.00\t57600.00\t58200.00\t58800.00\t59400.00\t60000.00\t60600.00\t61200.00\t61800.00\t62400.00\t63000.00\t63600.00\t64200.00\t64800.00\t65400.00\t66000.00\t66600.00\t67200.00\t67800.00\t68400.00\t69000.00\t69600.00\t70200.00\t70800.00\t71400.00\t72000.00\t72600.00\t73200.00\t73800.00\t74400.00\t75000.00\t75600.00\t76200.00\t76800.00\t77400.00\t78000.00\t78600.00\t79200.00\t79800.00\t80400.00\t81000.00\t81600.00\t82200.00\t82800.00\t83400.00\t84000.00\t84600.00\t85200.00\t85800.00\t86400.00]"  BeginIndexSearchUsingPreviousIndexResult=on  Table="[176.6\t168.8\t171.0\t162.4\t139.2\t135.7\t136.1\t126.4\t115.3\t119.1\t120.9\t112.9\t108.8\t108.4\t108.6\t115.7\t109.1\t110.1\t104.3\t102.4\t107.1\t108.6\t105.0\t101.7\t101.0\t100.5\t104.1\t105.9\t110.2\t113.1\t112.9\t122.1\t109.2\t120.3\t118.6\t122.6\t124.2\t134.1\t162.8\t189.0\t309.3\t319.3\t364.8\t346.9\t417.0\t276.3\t256.5\t386.4\t343.0\t281.6\t284.9\t297.7\t367.6\t344.5\t340.2\t401.7\t337.5\t290.1\t263.4\t283.0\t256.4\t264.4\t333.9\t339.9\t228.2\t258.4\t286.7\t337.2\t345.7\t283.4\t271.5\t301.9\t315.2\t222.7\t260.5\t314.4\t276.6\t251.0\t286.5\t277.6\t337.1\t293.1\t272.6\t264.0\t234.7\t266.6\t312.4\t300.4\t272.7\t275.3\t328.8\t303.7\t296.9\t271.1\t276.5\t287.6\t336.9\t310.5\t308.1\t352.7\t369.3\t416.5\t395.6\t425.3\t391.6\t343.9\t385.2\t411.7\t419.9\t433.6\t448.9\t437.5\t456.3\t466.2\t475.8\t478.2\t421.9\t455.4\t432.7\t434.7\t414.2\t380.6\t376.3\t380.7\t364.6\t365.6\t376.3\t400.0\t428.4\t382.9\t369.3\t440.8\t388.9\t372.9\t362.3\t328.6\t292.7\t286.7\t266.4\t263.2\t248.0\t239.3\t218.5\t190.8\t176.6]"  InternalRulePriority=Speed  RndMeth=Simplest  InputSameDT=on
  Magnitude-Angle to Complex1 : MagnitudeAngleToComplex
  Snubber3 : powerlib/Elements/Series RLC Branch  LConnTagsString=__new0  RConnTagsString=__new0  BranchType=R  Resistance=1e6  Inductance=1e-3  SetiL0=off  InitialCurrent=0  Capacitance=1e-6  Setx0=off  InitialVoltage=0  Measurements=None
      settings: SourceProductName=Simscape Electrical
  meas cur2 : powerlib/Measurements/Current Measurement  PhasorSimulation=on  OutputType=Complex  PSBequivalent=0
      settings: SourceProductName=Simscape Electrical
  Conn1 : PMIOPort  Side=Left
  Conn2 : PMIOPort  Port=2  Side=Right
  Out1 : Outport
  wires:
  meas cur2/1 -> Out1/1
  Clock/1 -> Load Data 1-D Lookup Table/1
  Magnitude-Angle to Complex1/1 -> Controlled Current Source4/1
  Load Data 1-D Lookup Table/1 -> Gain6/1
  Complex to Magnitude-Angle/1 -> Magnitude-Angle to Complex1/2
  Gain10/1 -> Magnitude-Angle to Complex1/1
  Gain6/1 -> Gain10/1
  [Vsec] -> Complex to Magnitude-Angle/1
  connections:
  Conn1/RConn1 -- meas cur2/LConn1
  Snubber3/LConn1 -- meas cur2/RConn1 -- Controlled Current Source4/RConn1
  Snubber3/RConn1 -- Controlled Current Source4/LConn1 -- Conn2/RConn1

== system power_microgrid_v5_battery/House 25 ==
  Clock : Clock
  Complex to Magnitude-Angle : ComplexToMagnitudeAngle  Output=Angle
  Controlled Current Source4 : powerlib/Electrical Sources/Controlled Current Source  Initialize=on  Source_Type=AC  Amplitude=0  Phase=0  Frequency=50  Measurements=None
      settings: SourceProductName=Simscape Electrical
  Gain10 : Gain  Gain=sqrt(2)
  Gain6 : Gain  Gain=-1/230
  Load Data 1-D Lookup Table : Lookup_n-D  NumberOfTableDimensions=1  BreakpointsForDimension1="[0.00\t600.00\t1200.00\t1800.00\t2400.00\t3000.00\t3600.00\t4200.00\t4800.00\t5400.00\t6000.00\t6600.00\t7200.00\t7800.00\t8400.00\t9000.00\t9600.00\t10200.00\t10800.00\t11400.00\t12000.00\t12600.00\t13200.00\t13800.00\t14400.00\t15000.00\t15600.00\t16200.00\t16800.00\t17400.00\t18000.00\t18600.00\t19200.00\t19800.00\t20400.00\t21000.00\t21600.00\t22200.00\t22800.00\t23400.00\t24000.00\t24600.00\t25200.00\t25800.00\t26400.00\t27000.00\t27600.00\t28200.00\t28800.00\t29400.00\t30000.00\t30600.00\t31200.00\t31800.00\t32400.00\t33000.00\t33600.00\t34200.00\t34800.00\t35400.00\t36000.00\t36600.00\t37200.00\t37800.00\t38400.00\t39000.00\t39600.00\t40200.00\t40800.00\t41400.00\t42000.00\t42600.00\t43200.00\t43800.00\t44400.00\t45000.00\t45600.00\t46200.00\t46800.00\t47400.00\t48000.00\t48600.00\t49200.00\t49800.00\t50400.00\t51000.00\t51600.00\t52200.00\t52800.00\t53400.00\t54000.00\t54600.00\t55200.00\t55800.00\t56400.00\t57000.00\t57600.00\t58200.00\t58800.00\t59400.00\t60000.00\t60600.00\t61200.00\t61800.00\t62400.00\t63000.00\t63600.00\t64200.00\t64800.00\t65400.00\t66000.00\t66600.00\t67200.00\t67800.00\t68400.00\t69000.00\t69600.00\t70200.00\t70800.00\t71400.00\t72000.00\t72600.00\t73200.00\t73800.00\t74400.00\t75000.00\t75600.00\t76200.00\t76800.00\t77400.00\t78000.00\t78600.00\t79200.00\t79800.00\t80400.00\t81000.00\t81600.00\t82200.00\t82800.00\t83400.00\t84000.00\t84600.00\t85200.00\t85800.00\t86400.00]"  BeginIndexSearchUsingPreviousIndexResult=on  Table="[176.6\t168.8\t171.0\t162.4\t139.2\t135.7\t136.1\t126.4\t115.3\t119.1\t120.9\t112.9\t108.8\t108.4\t108.6\t115.7\t109.1\t110.1\t104.3\t102.4\t107.1\t108.6\t105.0\t101.7\t101.0\t100.5\t104.1\t105.9\t110.2\t113.1\t112.9\t122.1\t109.2\t120.3\t118.6\t122.6\t124.2\t134.1\t162.8\t189.0\t309.3\t319.3\t364.8\t346.9\t417.0\t276.3\t256.5\t386.4\t343.0\t281.6\t284.9\t297.7\t367.6\t344.5\t340.2\t401.7\t337.5\t290.1\t263.4\t283.0\t256.4\t264.4\t333.9\t339.9\t228.2\t258.4\t286.7\t337.2\t345.7\t283.4\t271.5\t301.9\t315.2\t222.7\t260.5\t314.4\t276.6\t251.0\t286.5\t277.6\t337.1\t293.1\t272.6\t264.0\t234.7\t266.6\t312.4\t300.4\t272.7\t275.3\t328.8\t303.7\t296.9\t271.1\t276.5\t287.6\t336.9\t310.5\t308.1\t352.7\t369.3\t416.5\t395.6\t425.3\t391.6\t343.9\t385.2\t411.7\t419.9\t433.6\t448.9\t437.5\t456.3\t466.2\t475.8\t478.2\t421.9\t455.4\t432.7\t434.7\t414.2\t380.6\t376.3\t380.7\t364.6\t365.6\t376.3\t400.0\t428.4\t382.9\t369.3\t440.8\t388.9\t372.9\t362.3\t328.6\t292.7\t286.7\t266.4\t263.2\t248.0\t239.3\t218.5\t190.8\t176.6]"  InternalRulePriority=Speed  RndMeth=Simplest  InputSameDT=on
  Magnitude-Angle to Complex1 : MagnitudeAngleToComplex
  Snubber3 : powerlib/Elements/Series RLC Branch  LConnTagsString=__new0  RConnTagsString=__new0  BranchType=R  Resistance=1e6  Inductance=1e-3  SetiL0=off  InitialCurrent=0  Capacitance=1e-6  Setx0=off  InitialVoltage=0  Measurements=None
      settings: SourceProductName=Simscape Electrical
  meas cur2 : powerlib/Measurements/Current Measurement  PhasorSimulation=on  OutputType=Complex  PSBequivalent=0
      settings: SourceProductName=Simscape Electrical
  Conn1 : PMIOPort  Side=Left
  Conn2 : PMIOPort  Port=2  Side=Right
  Out1 : Outport
  wires:
  Magnitude-Angle to Complex1/1 -> Controlled Current Source4/1
  meas cur2/1 -> Out1/1
  Clock/1 -> Load Data 1-D Lookup Table/1
  Load Data 1-D Lookup Table/1 -> Gain6/1
  [Vsec] -> Complex to Magnitude-Angle/1
  Gain6/1 -> Gain10/1
  Gain10/1 -> Magnitude-Angle to Complex1/1
  Complex to Magnitude-Angle/1 -> Magnitude-Angle to Complex1/2
  connections:
  meas cur2/LConn1 -- Conn1/RConn1
  Snubber3/LConn1 -- Controlled Current Source4/RConn1 -- meas cur2/RConn1
  Snubber3/RConn1 -- Controlled Current Source4/LConn1 -- Conn2/RConn1
